simulink model "diagramaDEBlocosCompletoSubSystemsFinal"  (R2023a)
settings: Solver=VariableStepAuto  StartTime=0.0  StopTime=4500.0  RelTol=1e-3
values from neighbouring files (symbols this model uses):
  a1 = pi * (11 / 2).^2    [ConstantesCPQ23m.m]    (also in lugardasRaizes.m)
  a2 = 10 * 16    (= 160)    [ConstantesCPQ23m.m]    (also in lugardasRaizes.m)
  Alpha = Cv2/(2*a1*(sqrt(h2ss)))    [ConstantesCPQ23m.m]    (also in lugardasRaizes.m)
  B = Cv2/(2*a2*(sqrt(h2ss)))    [ConstantesCPQ23m.m]    (also in lugardasRaizes.m)
  bA2 = B*a2    [ConstantesCPQ23m.m]    (also in lugardasRaizes.m)
  Cv1 = 3.582    [ConstantesCPQ23m.m]    (also in lugardasRaizes.m)
  Cv2 = 2.869    [ConstantesCPQ23m.m]    (also in lugardasRaizes.m)
  F2 = 6.32    [ConstantesCPQ23m.m]    (also in lugardasRaizes.m)
  Gama = Cv1/(2*a1*(sqrt(h1ss)))    [ConstantesCPQ23m.m]    (also in lugardasRaizes.m)
  h1ss = sol(2)    [ConstantesCPQ23m.m]    (also in lugardasRaizes.m)
  h2ss = sol(1)    [ConstantesCPQ23m.m]    (also in lugardasRaizes.m)
  J = ((Alpha)/(B*a2*Gama))    [ConstantesCPQ23m.m]    (also in lugardasRaizes.m)
settings Model: Creator=Estudo  LastModifiedBy=Estudo

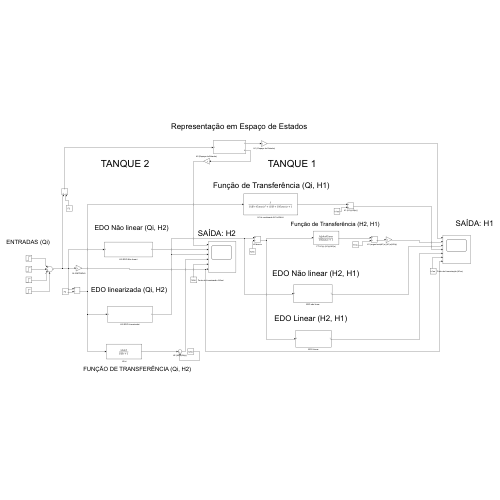
[thumbnail: Simulink's stored preview of the top-level diagram]
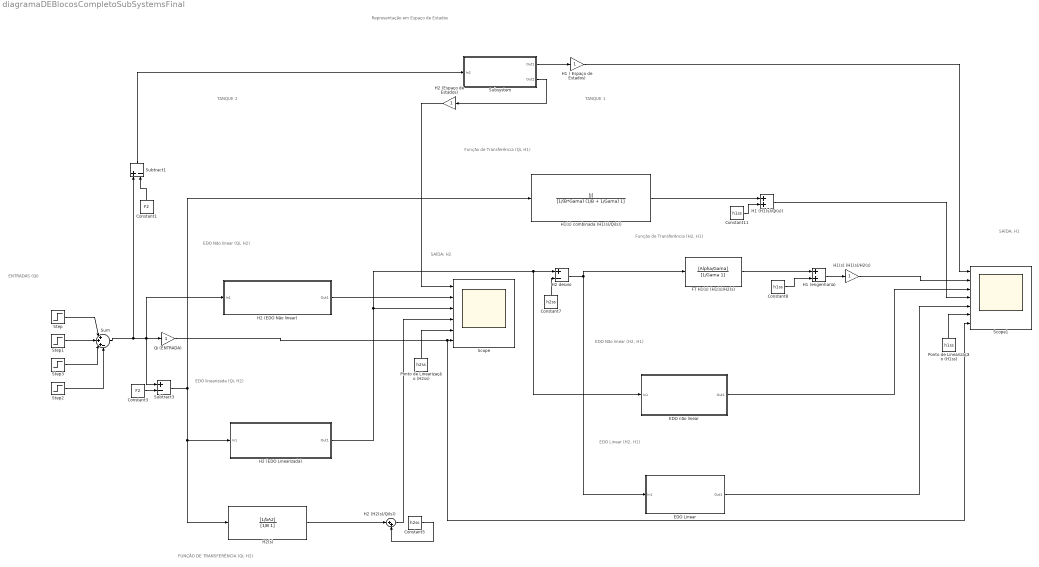
== system diagramaDEBlocosCompletoSubSystemsFinal ==
  note: Representação em Espaço de Estados
  note: Função de Transferência (H2, H1)
  note: TANQUE 1
  note: SAÍDA: H1
  note: ENTRADAS (Qi)
  note: EDO Linear (H2, H1)
  note: Função de Transferência (Qi, H1)
  note: FUNÇÃO DE TRANSFERÊNCIA (Qi, H2)
  note: EDO Não linear (H2, H1)
  note: EDO linearizada (Qi, H2)
  note: TANQUE 2
  note: SAÍDA: H2
  note: EDO Não linear (Qi, H2)
  Constant1 : Constant  Value=F2
  Constant11 : Constant  Value=h1ss
  Constant3 : Constant  Value=F2
  Constant5 : Constant  Value=h2ss
  Constant7 : Constant  Value=h2ss
  Constant8 : Constant  Value=h1ss
  EDO Linear : Subsystem
  EDO não linear : Subsystem
  FT H1(s) (H1(s)/H2(s) : TransferFcn  Numerator=[Alpha/Gama]  Denominator=[1/Gama 1]
  H1 ( Espaço de Estados) : Gain
  H1 (H1(s)/Qi(s)) : Sum
  H1 (engenharia) : Sum
  H1(s) (H1(s)/H2(s) : Gain
  H1(s) combinada (H1(s)/Qi(s)) : TransferFcn  Numerator=[J]  Denominator=[1/(B*Gama) (1/B + 1/Gama) 1]
  H2 (EDO Linearizada) : Subsystem
  H2 (EDO Não linear) : Subsystem
  H2 (Espaço de Estados) : Gain
  H2 (H2(s)/Qi(s)) : Sum  Inputs=|++
  H2 desvio : Sum  Inputs=+-
  H2(s) : TransferFcn  Numerator=[1/bA2]  Denominator=[1/B 1]
  Ponto de Linearização (H1ss) : Constant  Value=h1ss
  Ponto de Linearização (H2ss) : Constant  Value=h2ss
  Qi (ENTRADA) : Gain
  Scope : Scope  NumInputPorts=6
  Scope1 : Scope  NumInputPorts=7
  Step : Step  Time=0  After=6.32  SampleTime=0
  Step1 : Step  Time=1000  After=F2*0.1  SampleTime=0
  Step2 : Step  Time=3000  After=0.9*(6.32)  SampleTime=0
  Step3 : Step  Time=2000  After=F2*0.3  SampleTime=0
  Subsystem : Subsystem
  Subtract1 : Sum  Inputs=+-
  Subtract3 : Sum  Inputs=+-
  Sum : Sum  Inputs=|+++-
  wires:
  EDO Linear/1(Out1) -> Scope1/5
  H2 (EDO Linearizada)/1(Out1) -> EDO não linear/1(In1), H2 desvio/1, Scope/3
  H2 (EDO Não linear)/1(Out1) -> Scope/2
  H2(s)/1 -> H2 (H2(s)/Qi(s))/1
  H2 desvio/1 -> FT H1(s) (H1(s)/H2(s)/1, EDO Linear/1(In1)
  H1 (H1(s)/Qi(s))/1 -> Scope1/4
  Step1/1 -> Sum/2
  Constant3/1 -> Subtract3/2
  H2 (H2(s)/Qi(s))/1 -> Scope/4
  Constant5/1 -> H2 (H2(s)/Qi(s))/2
  Constant11/1 -> H1 (H1(s)/Qi(s))/2
  Step/1 -> Sum/1
  EDO não linear/1(Out1) -> Scope1/3
  H1(s) combinada (H1(s)/Qi(s))/1 -> H1 (H1(s)/Qi(s))/1
  FT H1(s) (H1(s)/H2(s)/1 -> H1 (engenharia)/1
  Constant8/1 -> H1 (engenharia)/2
  Sum/1 -> Qi (ENTRADA)/1, H2 (EDO Não linear)/1(In1), Subtract3/1, Subtract1/1
  Subtract3/1 -> H2(s)/1, H2 (EDO Linearizada)/1(In1), H1(s) combinada (H1(s)/Qi(s))/1
  Constant7/1 -> H2 desvio/2
  Ponto de Linearização (H2ss)/1 -> Scope/5
  Step2/1 -> Sum/4
  Step3/1 -> Sum/3
  Constant1/1 -> Subtract1/2
  H1 (engenharia)/1 -> H1(s) (H1(s)/H2(s)/1
  H1(s) (H1(s)/H2(s)/1 -> Scope1/2
  Subtract1/1 -> Subsystem/1(In2)
  Subsystem/1(Out1) -> H1 ( Espaço de Estados)/1
  H1 ( Espaço de Estados)/1 -> Scope1/1
  Subsystem/2(Out2) -> H2 (Espaço de Estados)/1
  H2 (Espaço de Estados)/1 -> Scope/1
  Ponto de Linearização (H1ss)/1 -> Scope1/6
  Qi (ENTRADA)/1 -> Scope/6, Scope1/7

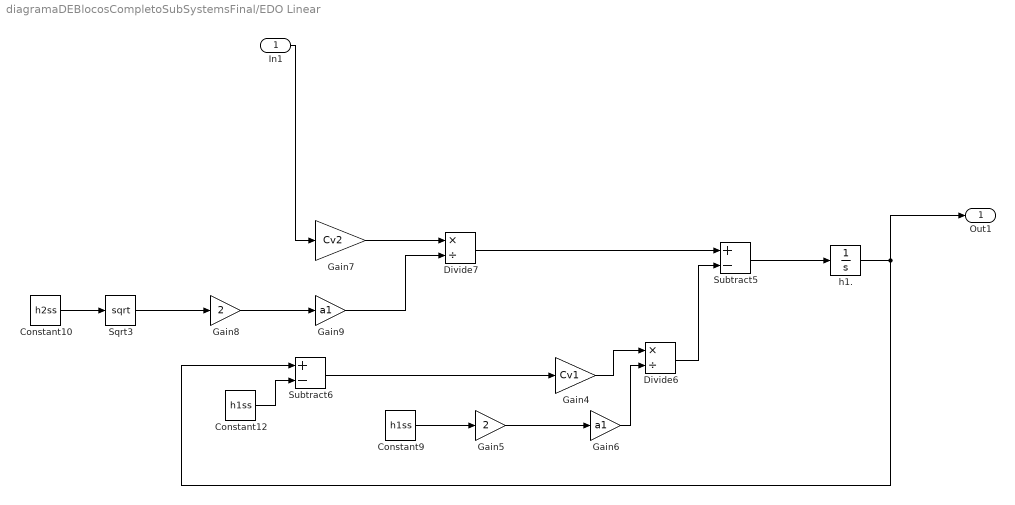
== system diagramaDEBlocosCompletoSubSystemsFinal/EDO Linear ==
  In1 : Inport
  Constant10 : Constant  Value=h2ss
  Constant12 : Constant  Value=h1ss
  Constant9 : Constant  Value=h1ss
  Divide6 : Product  Inputs=*/
  Divide7 : Product  Inputs=*/
  Gain4 : Gain  Gain=Cv1
  Gain5 : Gain  Gain=2
  Gain6 : Gain  Gain=a1
  Gain7 : Gain  Gain=Cv2
  Gain8 : Gain  Gain=2
  Gain9 : Gain  Gain=a1
  Sqrt3 : Sqrt
  Subtract5 : Sum  Inputs=+-
  Subtract6 : Sum  Inputs=+-
  h1. : Integrator  InitialCondition=h1ss
  Out1 : Outport
  wires:
  In1/1 -> Gain7/1
  Divide7/1 -> Subtract5/1
  Gain6/1 -> Divide6/2
  Constant9/1 -> Gain5/1
  Divide6/1 -> Subtract5/2
  Constant12/1 -> Subtract6/2
  Subtract6/1 -> Gain4/1
  Gain4/1 -> Divide6/1
  Gain7/1 -> Divide7/1
  Subtract5/1 -> h1./1
  Gain9/1 -> Divide7/2
  Gain8/1 -> Gain9/1
  Sqrt3/1 -> Gain8/1
  Gain5/1 -> Gain6/1
  Constant10/1 -> Sqrt3/1
  h1./1 -> Out1/1, Subtract6/1

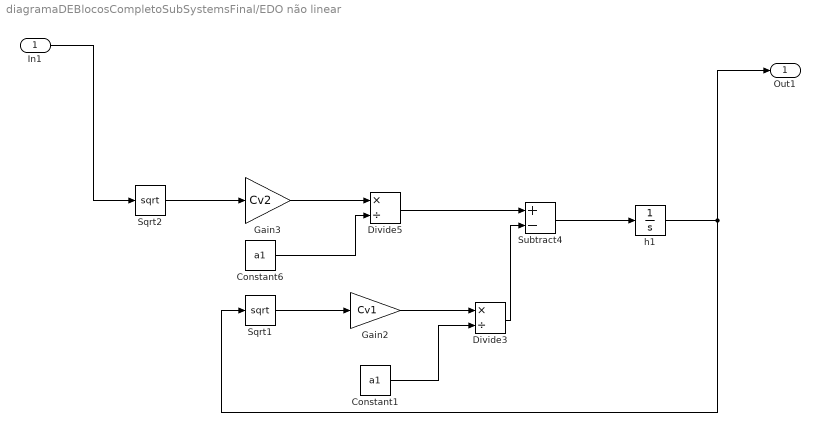
== system diagramaDEBlocosCompletoSubSystemsFinal/EDO não linear ==
  In1 : Inport
  Constant1 : Constant  Value=a1
  Constant6 : Constant  Value=a1
  Divide3 : Product  Inputs=*/
  Divide5 : Product  Inputs=*/
  Gain2 : Gain  Gain=Cv1
  Gain3 : Gain  Gain=Cv2
  Sqrt1 : Sqrt
  Sqrt2 : Sqrt
  Subtract4 : Sum  Inputs=+-
  h1 : Integrator  InitialCondition=h1ss
  Out1 : Outport
  wires:
  Divide3/1 -> Subtract4/2
  Constant6/1 -> Divide5/2
  Sqrt2/1 -> Gain3/1
  Gain2/1 -> Divide3/1
  Divide5/1 -> Subtract4/1
  Subtract4/1 -> h1/1
  Gain3/1 -> Divide5/1
  Sqrt1/1 -> Gain2/1
  h1/1 -> Out1/1, Sqrt1/1
  Constant1/1 -> Divide3/2
  In1/1 -> Sqrt2/1

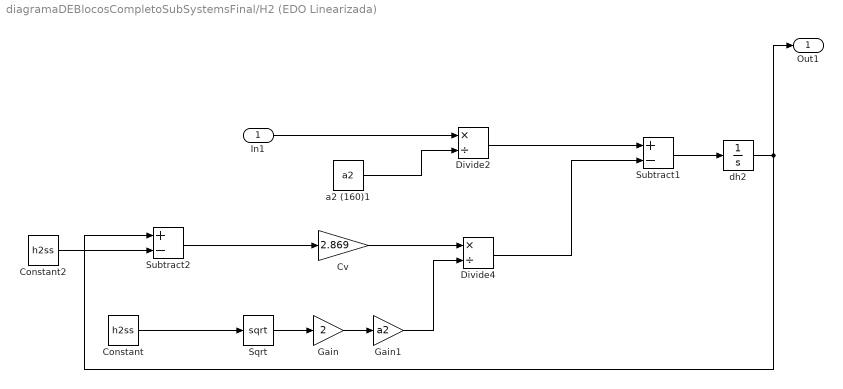
== system diagramaDEBlocosCompletoSubSystemsFinal/H2 (EDO Linearizada) ==
  In1 : Inport
  Constant : Constant  Value=h2ss
  Constant2 : Constant  Value=h2ss
  Cv : Gain  Gain=2.869
  Divide2 : Product  Inputs=*/
  Divide4 : Product  Inputs=*/
  Gain : Gain  Gain=2
  Gain1 : Gain  Gain=a2
  Sqrt : Sqrt
  Subtract1 : Sum  Inputs=+-
  Subtract2 : Sum  Inputs=+-
  a2 (160)1 : Constant  Value=a2
  dh2 : Integrator  InitialCondition=h2ss
  Out1 : Outport
  wires:
  Divide2/1 -> Subtract1/1
  Divide4/1 -> Subtract1/2
  dh2/1 -> Out1/1, Subtract2/1
  Constant/1 -> Sqrt/1
  Constant2/1 -> Subtract2/2
  Gain1/1 -> Divide4/2
  Subtract1/1 -> dh2/1
  Gain/1 -> Gain1/1
  Cv/1 -> Divide4/1
  a2 (160)1/1 -> Divide2/2
  Subtract2/1 -> Cv/1
  Sqrt/1 -> Gain/1
  In1/1 -> Divide2/1

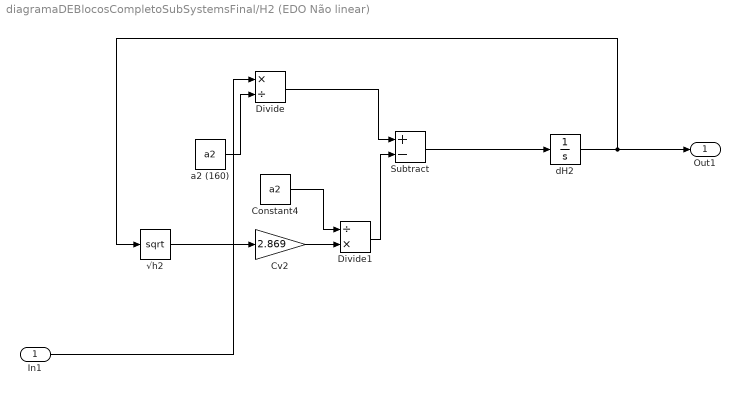
== system diagramaDEBlocosCompletoSubSystemsFinal/H2 (EDO Não linear) ==
  In1 : Inport
  Constant4 : Constant  Value=a2
  Cv2 : Gain  Gain=2.869
  Divide : Product  Inputs=*/
  Divide1 : Product  Inputs=/*
  Subtract : Sum  Inputs=+-
  a2 (160) : Constant  Value=a2
  dH2 : Integrator  InitialCondition=h2ss
  √h2 : Sqrt
  Out1 : Outport
  wires:
  Divide1/1 -> Subtract/2
  a2 (160)/1 -> Divide/2
  Cv2/1 -> Divide1/2
  Divide/1 -> Subtract/1
  Subtract/1 -> dH2/1
  √h2/1 -> Cv2/1
  dH2/1 -> √h2/1, Out1/1
  In1/1 -> Divide/1
  Constant4/1 -> Divide1/1

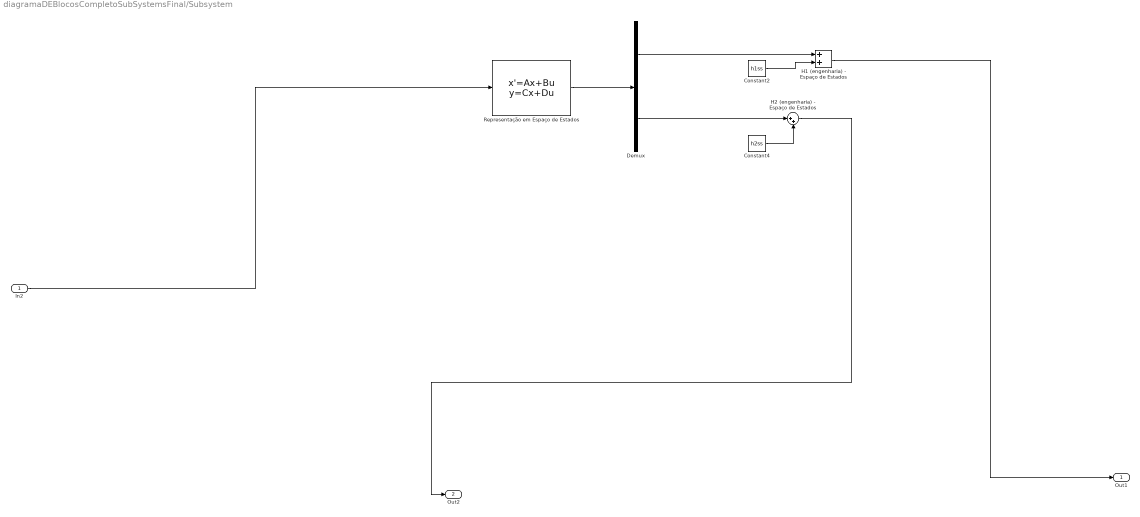
== system diagramaDEBlocosCompletoSubSystemsFinal/Subsystem ==
  In2 : Inport
  Constant2 : Constant  Value=h1ss
  Constant4 : Constant  Value=h2ss
  Demux : Demux  Outputs=2
  H1 (engenharia) - Espaço de Estados : Sum
  H2 (engenharia) - Espaço de Estados : Sum  Inputs=|++
  Representação em Espaço de Estados : StateSpace  A=[-Cv1/(2*a1*sqrt(h1ss)), Cv2/(2*a1*sqrt(h2ss)); 0, -Cv2/(2*a2*sqrt(h2ss))]  B=[0; 1/a2]  C=[1, 0; 0, 1]  D=[0; 0]  InitialCondition=0
  Out1 : Outport
  Out2 : Outport  Port=2
  wires:
  Representação em Espaço de Estados/1 -> Demux/1
  Demux/2 -> H2 (engenharia) - Espaço de Estados/1
  In2/1 -> Representação em Espaço de Estados/1
  Constant4/1 -> H2 (engenharia) - Espaço de Estados/2
  H1 (engenharia) - Espaço de Estados/1 -> Out1/1
  Constant2/1 -> H1 (engenharia) - Espaço de Estados/2
  Demux/1 -> H1 (engenharia) - Espaço de Estados/1
  H2 (engenharia) - Espaço de Estados/1 -> Out2/1
